simulink model "SIFT_final"  (R2015a)
settings: Solver=ode45  StartTime=0.0  StopTime=10.0  RelTol=1e-3
InitFcn:
  | %% DSPBuilder Start
  | alt_dspbuilder_update_model(bdroot)
  | %% DSPBuilder End
libraries: allblocks_alteradspbuilder2 x1826
(part 5 of 24)

== system SIFT_final/SIFT/Calculate_descriptor/hist_bin/Line_buffer_5x5_1 ==
  dataIn : Inport
  clken : Inport  Port=2
  Delay : allblocks_alteradspbuilder2/Delay  pipeline=1  pipeline_display=1  ClockPhase=1  use_ena=on  use_sclr=off  allowFloatingPointOverride=on  logOutputs=off  logFile=C:\Users\ASUS\Desktop\final_sift_fpga\tb_SIFT_detection_feature\SIFT%5Fdetection%5Ffeature_calculate%5Fdescriptor_hist%5Fbin_Line%5Fbuffer%5F5x5%5F1_Delay.fixedpointlog  use_init=off  reset_value=1
  Delay1 : allblocks_alteradspbuilder2/Delay  pipeline=1  pipeline_display=1  ClockPhase=1  use_ena=on  use_sclr=off  allowFloatingPointOverride=on  logOutputs=off  logFile=C:\Users\ASUS\Desktop\final_sift_fpga\tb_SIFT_detection_feature\SIFT%5Fdetection%5Ffeature_calculate%5Fdescriptor_hist%5Fbin_Line%5Fbuffer%5F5x5%5F1_Delay1.fixedpointlog  use_init=off  reset_value=1
  Delay10 : allblocks_alteradspbuilder2/Delay  pipeline=1  pipeline_display=1  ClockPhase=1  use_ena=on  use_sclr=off  allowFloatingPointOverride=on  logOutputs=off  logFile=C:\Users\ASUS\Desktop\final_sift_fpga\tb_SIFT_detection_feature\SIFT%5Fdetection%5Ffeature_calculate%5Fdescriptor_hist%5Fbin_Line%5Fbuffer%5F5x5%5F1_Delay10.fixedpointlog  use_init=off  reset_value=1
  Delay11 : allblocks_alteradspbuilder2/Delay  pipeline=1  pipeline_display=1  ClockPhase=1  use_ena=on  use_sclr=off  allowFloatingPointOverride=on  logOutputs=off  logFile=C:\Users\ASUS\Desktop\final_sift_fpga\tb_SIFT_detection_feature\SIFT%5Fdetection%5Ffeature_calculate%5Fdescriptor_hist%5Fbin_Line%5Fbuffer%5F5x5%5F1_Delay11.fixedpointlog  use_init=off  reset_value=1
  Delay12 : allblocks_alteradspbuilder2/Delay  pipeline=1  pipeline_display=1  ClockPhase=1  use_ena=on  use_sclr=off  allowFloatingPointOverride=on  logOutputs=off  logFile=C:\Users\ASUS\Desktop\final_sift_fpga\tb_SIFT_detection_feature\SIFT%5Fdetection%5Ffeature_calculate%5Fdescriptor_hist%5Fbin_Line%5Fbuffer%5F5x5%5F1_Delay12.fixedpointlog  use_init=off  reset_value=1
  Delay13 : allblocks_alteradspbuilder2/Delay  pipeline=1  pipeline_display=1  ClockPhase=1  use_ena=on  use_sclr=off  allowFloatingPointOverride=on  logOutputs=off  logFile=C:\Users\ASUS\Desktop\final_sift_fpga\tb_SIFT_detection_feature\SIFT%5Fdetection%5Ffeature_calculate%5Fdescriptor_hist%5Fbin_Line%5Fbuffer%5F5x5%5F1_Delay13.fixedpointlog  use_init=off  reset_value=1
  Delay14 : allblocks_alteradspbuilder2/Delay  pipeline=1  pipeline_display=1  ClockPhase=1  use_ena=on  use_sclr=off  allowFloatingPointOverride=on  logOutputs=off  logFile=C:\Users\ASUS\Desktop\final_sift_fpga\tb_SIFT_detection_feature\SIFT%5Fdetection%5Ffeature_calculate%5Fdescriptor_hist%5Fbin_Line%5Fbuffer%5F5x5%5F1_Delay14.fixedpointlog  use_init=off  reset_value=1
  Delay15 : allblocks_alteradspbuilder2/Delay  pipeline=1  pipeline_display=1  ClockPhase=1  use_ena=on  use_sclr=off  allowFloatingPointOverride=on  logOutputs=off  logFile=C:\Users\ASUS\Desktop\final_sift_fpga\tb_SIFT_detection_feature\SIFT%5Fdetection%5Ffeature_calculate%5Fdescriptor_hist%5Fbin_Line%5Fbuffer%5F5x5%5F1_Delay15.fixedpointlog  use_init=off  reset_value=1
  Delay16 : allblocks_alteradspbuilder2/Delay  pipeline=1  pipeline_display=1  ClockPhase=1  use_ena=on  use_sclr=off  allowFloatingPointOverride=on  logOutputs=off  logFile=C:\Users\ASUS\Desktop\final_sift_fpga\tb_SIFT_detection_feature\SIFT%5Fdetection%5Ffeature_calculate%5Fdescriptor_hist%5Fbin_Line%5Fbuffer%5F5x5%5F1_Delay16.fixedpointlog  use_init=off  reset_value=1
  Delay17 : allblocks_alteradspbuilder2/Delay  pipeline=1  pipeline_display=1  ClockPhase=1  use_ena=on  use_sclr=off  allowFloatingPointOverride=on  logOutputs=off  logFile=C:\Users\ASUS\Desktop\final_sift_fpga\tb_SIFT_detection_feature\SIFT%5Fdetection%5Ffeature_calculate%5Fdescriptor_hist%5Fbin_Line%5Fbuffer%5F5x5%5F1_Delay17.fixedpointlog  use_init=off  reset_value=1
  Delay18 : allblocks_alteradspbuilder2/Delay  pipeline=1  pipeline_display=1  ClockPhase=1  use_ena=on  use_sclr=off  allowFloatingPointOverride=on  logOutputs=off  logFile=C:\Users\ASUS\Desktop\final_sift_fpga\tb_SIFT_detection_feature\SIFT%5Fdetection%5Ffeature_calculate%5Fdescriptor_hist%5Fbin_Line%5Fbuffer%5F5x5%5F1_Delay18.fixedpointlog  use_init=off  reset_value=1
  Delay19 : allblocks_alteradspbuilder2/Delay  pipeline=1  pipeline_display=1  ClockPhase=1  use_ena=on  use_sclr=off  allowFloatingPointOverride=on  logOutputs=off  logFile=C:\Users\ASUS\Desktop\final_sift_fpga\tb_SIFT_detection_feature\SIFT%5Fdetection%5Ffeature_calculate%5Fdescriptor_hist%5Fbin_Line%5Fbuffer%5F5x5%5F1_Delay19.fixedpointlog  use_init=off  reset_value=1
  Delay2 : allblocks_alteradspbuilder2/Delay  pipeline=1  pipeline_display=1  ClockPhase=1  use_ena=on  use_sclr=off  allowFloatingPointOverride=on  logOutputs=off  logFile=C:\Users\ASUS\Desktop\final_sift_fpga\tb_SIFT_detection_feature\SIFT%5Fdetection%5Ffeature_calculate%5Fdescriptor_hist%5Fbin_Line%5Fbuffer%5F5x5%5F1_Delay2.fixedpointlog  use_init=off  reset_value=1
  Delay20 : allblocks_alteradspbuilder2/Delay  pipeline=1  pipeline_display=1  ClockPhase=1  use_ena=on  use_sclr=off  allowFloatingPointOverride=on  logOutputs=off  logFile=C:\Users\ASUS\Desktop\final_sift_fpga\tb_SIFT_detection_feature\SIFT%5Fdetection%5Ffeature_calculate%5Fdescriptor_hist%5Fbin_Line%5Fbuffer%5F5x5%5F1_Delay20.fixedpointlog  use_init=off  reset_value=1
  Delay21 : allblocks_alteradspbuilder2/Delay  pipeline=16  pipeline_display=16  ClockPhase=1  use_ena=on  use_sclr=off  allowFloatingPointOverride=on  logOutputs=off  logFile=C:\Users\ASUS\Desktop\final_sift_fpga\tb_SIFT_detection_feature\SIFT%5Fdetection%5Ffeature_calculate%5Fdescriptor_hist%5Fbin_Line%5Fbuffer%5F5x5%5F1_Delay21.fixedpointlog  use_init=off  reset_value=1
  Delay22 : allblocks_alteradspbuilder2/Delay  pipeline=16  pipeline_display=16  ClockPhase=1  use_ena=on  use_sclr=off  allowFloatingPointOverride=on  logOutputs=off  logFile=C:\Users\ASUS\Desktop\final_sift_fpga\tb_SIFT_detection_feature\SIFT%5Fdetection%5Ffeature_calculate%5Fdescriptor_hist%5Fbin_Line%5Fbuffer%5F5x5%5F1_Delay22.fixedpointlog  use_init=off  reset_value=1
  Delay23 : allblocks_alteradspbuilder2/Delay  pipeline=16  pipeline_display=16  ClockPhase=1  use_ena=on  use_sclr=off  allowFloatingPointOverride=on  logOutputs=off  logFile=C:\Users\ASUS\Desktop\final_sift_fpga\tb_SIFT_detection_feature\SIFT%5Fdetection%5Ffeature_calculate%5Fdescriptor_hist%5Fbin_Line%5Fbuffer%5F5x5%5F1_Delay23.fixedpointlog  use_init=off  reset_value=1
  Delay24 : allblocks_alteradspbuilder2/Delay  pipeline=16  pipeline_display=16  ClockPhase=1  use_ena=on  use_sclr=off  allowFloatingPointOverride=on  logOutputs=off  logFile=C:\Users\ASUS\Desktop\final_sift_fpga\tb_SIFT_detection_feature\SIFT%5Fdetection%5Ffeature_calculate%5Fdescriptor_hist%5Fbin_Line%5Fbuffer%5F5x5%5F1_Delay24.fixedpointlog  use_init=off  reset_value=1
  Delay25 : allblocks_alteradspbuilder2/Delay  pipeline=16  pipeline_display=16  ClockPhase=1  use_ena=on  use_sclr=off  allowFloatingPointOverride=on  logOutputs=off  logFile=C:\Users\ASUS\Desktop\final_sift_fpga\tb_SIFT_detection_feature\SIFT%5Fdetection%5Ffeature_calculate%5Fdescriptor_hist%5Fbin_Line%5Fbuffer%5F5x5%5F1_Delay25.fixedpointlog  use_init=off  reset_value=1
  Delay26 : allblocks_alteradspbuilder2/Delay  pipeline=16  pipeline_display=16  ClockPhase=1  use_ena=on  use_sclr=off  allowFloatingPointOverride=on  logOutputs=off  logFile=C:\Users\ASUS\Desktop\final_sift_fpga\tb_SIFT_detection_feature\SIFT%5Fdetection%5Ffeature_calculate%5Fdescriptor_hist%5Fbin_Line%5Fbuffer%5F5x5%5F1_Delay26.fixedpointlog  use_init=off  reset_value=1
  Delay27 : allblocks_alteradspbuilder2/Delay  pipeline=16  pipeline_display=16  ClockPhase=1  use_ena=on  use_sclr=off  allowFloatingPointOverride=on  logOutputs=off  logFile=C:\Users\ASUS\Desktop\final_sift_fpga\tb_SIFT_detection_feature\SIFT%5Fdetection%5Ffeature_calculate%5Fdescriptor_hist%5Fbin_Line%5Fbuffer%5F5x5%5F1_Delay27.fixedpointlog  use_init=off  reset_value=1
  Delay28 : allblocks_alteradspbuilder2/Delay  pipeline=16  pipeline_display=16  ClockPhase=1  use_ena=on  use_sclr=off  allowFloatingPointOverride=on  logOutputs=off  logFile=C:\Users\ASUS\Desktop\final_sift_fpga\tb_SIFT_detection_feature\SIFT%5Fdetection%5Ffeature_calculate%5Fdescriptor_hist%5Fbin_Line%5Fbuffer%5F5x5%5F1_Delay28.fixedpointlog  use_init=off  reset_value=1
  Delay29 : allblocks_alteradspbuilder2/Delay  pipeline=16  pipeline_display=16  ClockPhase=1  use_ena=on  use_sclr=off  allowFloatingPointOverride=on  logOutputs=off  logFile=C:\Users\ASUS\Desktop\final_sift_fpga\tb_SIFT_detection_feature\SIFT%5Fdetection%5Ffeature_calculate%5Fdescriptor_hist%5Fbin_Line%5Fbuffer%5F5x5%5F1_Delay29.fixedpointlog  use_init=off  reset_value=1
  Delay3 : allblocks_alteradspbuilder2/Delay  pipeline=1  pipeline_display=1  ClockPhase=1  use_ena=on  use_sclr=off  allowFloatingPointOverride=on  logOutputs=off  logFile=C:\Users\ASUS\Desktop\final_sift_fpga\tb_SIFT_detection_feature\SIFT%5Fdetection%5Ffeature_calculate%5Fdescriptor_hist%5Fbin_Line%5Fbuffer%5F5x5%5F1_Delay3.fixedpointlog  use_init=off  reset_value=1
  Delay30 : allblocks_alteradspbuilder2/Delay  pipeline=16  pipeline_display=16  ClockPhase=1  use_ena=on  use_sclr=off  allowFloatingPointOverride=on  logOutputs=off  logFile=C:\Users\ASUS\Desktop\final_sift_fpga\tb_SIFT_detection_feature\SIFT%5Fdetection%5Ffeature_calculate%5Fdescriptor_hist%5Fbin_Line%5Fbuffer%5F5x5%5F1_Delay30.fixedpointlog  use_init=off  reset_value=1
  Delay31 : allblocks_alteradspbuilder2/Delay  pipeline=16  pipeline_display=16  ClockPhase=1  use_ena=on  use_sclr=off  allowFloatingPointOverride=on  logOutputs=off  logFile=C:\Users\ASUS\Desktop\final_sift_fpga\tb_SIFT_detection_feature\SIFT%5Fdetection%5Ffeature_calculate%5Fdescriptor_hist%5Fbin_Line%5Fbuffer%5F5x5%5F1_Delay31.fixedpointlog  use_init=off  reset_value=1
  Delay32 : allblocks_alteradspbuilder2/Delay  pipeline=16  pipeline_display=16  ClockPhase=1  use_ena=on  use_sclr=off  allowFloatingPointOverride=on  logOutputs=off  logFile=C:\Users\ASUS\Desktop\final_sift_fpga\tb_SIFT_detection_feature\SIFT%5Fdetection%5Ffeature_calculate%5Fdescriptor_hist%5Fbin_Line%5Fbuffer%5F5x5%5F1_Delay32.fixedpointlog  use_init=off  reset_value=1
  Delay33 : allblocks_alteradspbuilder2/Delay  pipeline=16  pipeline_display=16  ClockPhase=1  use_ena=on  use_sclr=off  allowFloatingPointOverride=on  logOutputs=off  logFile=C:\Users\ASUS\Desktop\final_sift_fpga\tb_SIFT_detection_feature\SIFT%5Fdetection%5Ffeature_calculate%5Fdescriptor_hist%5Fbin_Line%5Fbuffer%5F5x5%5F1_Delay33.fixedpointlog  use_init=off  reset_value=1
  Delay34 : allblocks_alteradspbuilder2/Delay  pipeline=16  pipeline_display=16  ClockPhase=1  use_ena=on  use_sclr=off  allowFloatingPointOverride=on  logOutputs=off  logFile=C:\Users\ASUS\Desktop\final_sift_fpga\tb_SIFT_detection_feature\SIFT%5Fdetection%5Ffeature_calculate%5Fdescriptor_hist%5Fbin_Line%5Fbuffer%5F5x5%5F1_Delay34.fixedpointlog  use_init=off  reset_value=1
  Delay35 : allblocks_alteradspbuilder2/Delay  pipeline=16  pipeline_display=16  ClockPhase=1  use_ena=on  use_sclr=off  allowFloatingPointOverride=on  logOutputs=off  logFile=C:\Users\ASUS\Desktop\final_sift_fpga\tb_SIFT_detection_feature\SIFT%5Fdetection%5Ffeature_calculate%5Fdescriptor_hist%5Fbin_Line%5Fbuffer%5F5x5%5F1_Delay35.fixedpointlog  use_init=off  reset_value=1
  Delay36 : allblocks_alteradspbuilder2/Delay  pipeline=16  pipeline_display=16  ClockPhase=1  use_ena=on  use_sclr=off  allowFloatingPointOverride=on  logOutputs=off  logFile=C:\Users\ASUS\Desktop\final_sift_fpga\tb_SIFT_detection_feature\SIFT%5Fdetection%5Ffeature_calculate%5Fdescriptor_hist%5Fbin_Line%5Fbuffer%5F5x5%5F1_Delay36.fixedpointlog  use_init=off  reset_value=1
  Delay37 : allblocks_alteradspbuilder2/Delay  pipeline=16  pipeline_display=16  ClockPhase=1  use_ena=on  use_sclr=off  allowFloatingPointOverride=on  logOutputs=off  logFile=C:\Users\ASUS\Desktop\final_sift_fpga\tb_SIFT_detection_feature\SIFT%5Fdetection%5Ffeature_calculate%5Fdescriptor_hist%5Fbin_Line%5Fbuffer%5F5x5%5F1_Delay37.fixedpointlog  use_init=off  reset_value=1
  Delay38 : allblocks_alteradspbuilder2/Delay  pipeline=16  pipeline_display=16  ClockPhase=1  use_ena=on  use_sclr=off  allowFloatingPointOverride=on  logOutputs=off  logFile=C:\Users\ASUS\Desktop\final_sift_fpga\tb_SIFT_detection_feature\SIFT%5Fdetection%5Ffeature_calculate%5Fdescriptor_hist%5Fbin_Line%5Fbuffer%5F5x5%5F1_Delay38.fixedpointlog  use_init=off  reset_value=1
  Delay39 : allblocks_alteradspbuilder2/Delay  pipeline=16  pipeline_display=16  ClockPhase=1  use_ena=on  use_sclr=off  allowFloatingPointOverride=on  logOutputs=off  logFile=C:\Users\ASUS\Desktop\final_sift_fpga\tb_SIFT_detection_feature\SIFT%5Fdetection%5Ffeature_calculate%5Fdescriptor_hist%5Fbin_Line%5Fbuffer%5F5x5%5F1_Delay39.fixedpointlog  use_init=off  reset_value=1
  Delay4 : allblocks_alteradspbuilder2/Delay  pipeline=1  pipeline_display=1  ClockPhase=1  use_ena=on  use_sclr=off  allowFloatingPointOverride=on  logOutputs=off  logFile=C:\Users\ASUS\Desktop\final_sift_fpga\tb_SIFT_detection_feature\SIFT%5Fdetection%5Ffeature_calculate%5Fdescriptor_hist%5Fbin_Line%5Fbuffer%5F5x5%5F1_Delay4.fixedpointlog  use_init=off  reset_value=1
  Delay40 : allblocks_alteradspbuilder2/Delay  pipeline=16  pipeline_display=16  ClockPhase=1  use_ena=on  use_sclr=off  allowFloatingPointOverride=on  logOutputs=off  logFile=C:\Users\ASUS\Desktop\final_sift_fpga\tb_SIFT_detection_feature\SIFT%5Fdetection%5Ffeature_calculate%5Fdescriptor_hist%5Fbin_Line%5Fbuffer%5F5x5%5F1_Delay40.fixedpointlog  use_init=off  reset_value=1
  Delay41 : allblocks_alteradspbuilder2/Delay  pipeline=16  pipeline_display=16  ClockPhase=1  use_ena=on  use_sclr=off  allowFloatingPointOverride=on  logOutputs=off  logFile=C:\Users\ASUS\Desktop\final_sift_fpga\tb_SIFT_detection_feature\SIFT%5Fdetection%5Ffeature_calculate%5Fdescriptor_hist%5Fbin_Line%5Fbuffer%5F5x5%5F1_Delay41.fixedpointlog  use_init=off  reset_value=1
  Delay42 : allblocks_alteradspbuilder2/Delay  pipeline=16  pipeline_display=16  ClockPhase=1  use_ena=on  use_sclr=off  allowFloatingPointOverride=on  logOutputs=off  logFile=C:\Users\ASUS\Desktop\final_sift_fpga\tb_SIFT_detection_feature\SIFT%5Fdetection%5Ffeature_calculate%5Fdescriptor_hist%5Fbin_Line%5Fbuffer%5F5x5%5F1_Delay42.fixedpointlog  use_init=off  reset_value=1
  Delay43 : allblocks_alteradspbuilder2/Delay  pipeline=16  pipeline_display=16  ClockPhase=1  use_ena=on  use_sclr=off  allowFloatingPointOverride=on  logOutputs=off  logFile=C:\Users\ASUS\Desktop\final_sift_fpga\tb_SIFT_detection_feature\SIFT%5Fdetection%5Ffeature_calculate%5Fdescriptor_hist%5Fbin_Line%5Fbuffer%5F5x5%5F1_Delay43.fixedpointlog  use_init=off  reset_value=1
  Delay44 : allblocks_alteradspbuilder2/Delay  pipeline=16  pipeline_display=16  ClockPhase=1  use_ena=on  use_sclr=off  allowFloatingPointOverride=on  logOutputs=off  logFile=C:\Users\ASUS\Desktop\final_sift_fpga\tb_SIFT_detection_feature\SIFT%5Fdetection%5Ffeature_calculate%5Fdescriptor_hist%5Fbin_Line%5Fbuffer%5F5x5%5F1_Delay44.fixedpointlog  use_init=off  reset_value=1
  Delay45 : allblocks_alteradspbuilder2/Delay  pipeline=16  pipeline_display=16  ClockPhase=1  use_ena=on  use_sclr=off  allowFloatingPointOverride=on  logOutputs=off  logFile=C:\Users\ASUS\Desktop\final_sift_fpga\tb_SIFT_detection_feature\SIFT%5Fdetection%5Ffeature_calculate%5Fdescriptor_hist%5Fbin_Line%5Fbuffer%5F5x5%5F1_Delay45.fixedpointlog  use_init=off  reset_value=1
  Delay5 : allblocks_alteradspbuilder2/Delay  pipeline=1  pipeline_display=1  ClockPhase=1  use_ena=on  use_sclr=off  allowFloatingPointOverride=on  logOutputs=off  logFile=C:\Users\ASUS\Desktop\final_sift_fpga\tb_SIFT_detection_feature\SIFT%5Fdetection%5Ffeature_calculate%5Fdescriptor_hist%5Fbin_Line%5Fbuffer%5F5x5%5F1_Delay5.fixedpointlog  use_init=off  reset_value=1
  Delay6 : allblocks_alteradspbuilder2/Delay  pipeline=1  pipeline_display=1  ClockPhase=1  use_ena=on  use_sclr=off  allowFloatingPointOverride=on  logOutputs=off  logFile=C:\Users\ASUS\Desktop\final_sift_fpga\tb_SIFT_detection_feature\SIFT%5Fdetection%5Ffeature_calculate%5Fdescriptor_hist%5Fbin_Line%5Fbuffer%5F5x5%5F1_Delay6.fixedpointlog  use_init=off  reset_value=1
  Delay7 : allblocks_alteradspbuilder2/Delay  pipeline=1  pipeline_display=1  ClockPhase=1  use_ena=on  use_sclr=off  allowFloatingPointOverride=on  logOutputs=off  logFile=C:\Users\ASUS\Desktop\final_sift_fpga\tb_SIFT_detection_feature\SIFT%5Fdetection%5Ffeature_calculate%5Fdescriptor_hist%5Fbin_Line%5Fbuffer%5F5x5%5F1_Delay7.fixedpointlog  use_init=off  reset_value=1
  Delay8 : allblocks_alteradspbuilder2/Delay  pipeline=1  pipeline_display=1  ClockPhase=1  use_ena=on  use_sclr=off  allowFloatingPointOverride=on  logOutputs=off  logFile=C:\Users\ASUS\Desktop\final_sift_fpga\tb_SIFT_detection_feature\SIFT%5Fdetection%5Ffeature_calculate%5Fdescriptor_hist%5Fbin_Line%5Fbuffer%5F5x5%5F1_Delay8.fixedpointlog  use_init=off  reset_value=1
  Delay9 : allblocks_alteradspbuilder2/Delay  pipeline=1  pipeline_display=1  ClockPhase=1  use_ena=on  use_sclr=off  allowFloatingPointOverride=on  logOutputs=off  logFile=C:\Users\ASUS\Desktop\final_sift_fpga\tb_SIFT_detection_feature\SIFT%5Fdetection%5Ffeature_calculate%5Fdescriptor_hist%5Fbin_Line%5Fbuffer%5F5x5%5F1_Delay9.fixedpointlog  use_init=off  reset_value=1
  Memory Delay : allblocks_alteradspbuilder2/Memory Delay  BusType=Unsigned Integer  bwl=8  bwr=0  pipeline=636  pipeline_display=636  ram_type=AUTO  use_ena=on  use_sclr=off  allowFloatingPointOverride=on  logOutputs=off  logFile=C:\Users\ASUS\Desktop\final_sift_fpga\tb_SIFT_detection_feature\SIFT%5Fdetection%5Ffeature_calculate%5Fdescriptor_hist%5Fbin_Line%5Fbuffer%5F5x5%5F1_Memory+Delay.fixedpointlog
  Memory Delay1 : allblocks_alteradspbuilder2/Memory Delay  BusType=Unsigned Integer  bwl=8  bwr=0  pipeline=636  pipeline_display=636  ram_type=AUTO  use_ena=on  use_sclr=off  allowFloatingPointOverride=on  logOutputs=off  logFile=C:\Users\ASUS\Desktop\final_sift_fpga\tb_SIFT_detection_feature\SIFT%5Fdetection%5Ffeature_calculate%5Fdescriptor_hist%5Fbin_Line%5Fbuffer%5F5x5%5F1_Memory+Delay1.fixedpointlog
  Memory Delay2 : allblocks_alteradspbuilder2/Memory Delay  BusType=Unsigned Integer  bwl=8  bwr=0  pipeline=636  pipeline_display=636  ram_type=AUTO  use_ena=on  use_sclr=off  allowFloatingPointOverride=on  logOutputs=off  logFile=C:\Users\ASUS\Desktop\final_sift_fpga\tb_SIFT_detection_feature\SIFT%5Fdetection%5Ffeature_calculate%5Fdescriptor_hist%5Fbin_Line%5Fbuffer%5F5x5%5F1_Memory+Delay2.fixedpointlog
  Memory Delay3 : allblocks_alteradspbuilder2/Memory Delay  BusType=Unsigned Integer  bwl=8  bwr=0  pipeline=636  pipeline_display=636  ram_type=AUTO  use_ena=on  use_sclr=off  allowFloatingPointOverride=on  logOutputs=off  logFile=C:\Users\ASUS\Desktop\final_sift_fpga\tb_SIFT_detection_feature\SIFT%5Fdetection%5Ffeature_calculate%5Fdescriptor_hist%5Fbin_Line%5Fbuffer%5F5x5%5F1_Memory+Delay3.fixedpointlog
  Out00 : Outport
  Out01 : Outport  Port=2
  Out02 : Outport  Port=3
  Out03 : Outport  Port=4
  Out04 : Outport  Port=5
  Out10 : Outport  Port=6
  Out11 : Outport  Port=7
  Out12 : Outport  Port=8
  Out13 : Outport  Port=9
  Out14 : Outport  Port=10
  Out20 : Outport  Port=11
  Out21 : Outport  Port=12
  Out22 : Outport  Port=13
  Out23 : Outport  Port=14
  Out24 : Outport  Port=15
  Out30 : Outport  Port=16
  Out31 : Outport  Port=17
  Out32 : Outport  Port=18
  Out33 : Outport  Port=19
  Out34 : Outport  Port=20
  Out40 : Outport  Port=21
  Out41 : Outport  Port=22
  Out42 : Outport  Port=23
  Out43 : Outport  Port=24
  Out44 : Outport  Port=25
  wires:
  [clken] -> Delay11/2
  Delay11/1 -> [data_23], Delay12/1
  [clken] -> Delay12/2
  [clken] -> Delay10/2
  Delay8/1 -> Memory Delay1/1, [data_14]
  [clken] -> Memory Delay1/2
  Delay9/1 -> [data_21], Delay10/1
  Memory Delay1/1 -> [data_20], Delay9/1
  Delay10/1 -> [data_22], Delay11/1
  [clken] -> Delay9/2
  [clken] -> Delay4/2
  Delay/1 -> [data_00], Delay1/1
  [clken] -> Delay1/2
  [clken] -> Delay/2
  [data_in] -> Delay/1
  [clken] -> Delay2/2
  Delay2/1 -> [data_02], Delay3/1
  Delay1/1 -> [data_01], Delay2/1
  [clken] -> Delay3/2
  clken/1 -> [clken]
  dataIn/1 -> [data_in]
  Delay4/1 -> Memory Delay/1, [data_04]
  [clken] -> Memory Delay/2
  Delay12/1 -> [data_24], Memory Delay2/1
  [clken] -> Memory Delay2/2
  Memory Delay2/1 -> [data_30], Delay16/1
  [clken] -> Delay16/2
  [clken] -> Delay14/2
  [clken] -> Delay15/2
  [clken] -> Memory Delay3/2
  Delay17/1 -> [data_32], Delay18/1
  Delay18/1 -> [data_33], Delay19/1
  Memory Delay3/1 -> [data_40], Delay20/1
  [clken] -> Delay20/2
  [clken] -> Delay19/2
  Delay13/1 -> [data_42], Delay14/1
  Delay19/1 -> Memory Delay3/1, [data_34]
  Delay14/1 -> [data_43], Delay15/1
  Delay15/1 -> [data_44]
  [clken] -> Delay17/2
  [clken] -> Delay18/2
  [clken] -> Delay13/2
  Delay16/1 -> [data_31], Delay17/1
  Delay20/1 -> [data_41], Delay13/1
  Memory Delay/1 -> [data_10], Delay5/1
  [clken] -> Delay7/2
  [clken] -> Delay6/2
  Delay5/1 -> [data_11], Delay6/1
  [clken] -> Delay8/2
  [clken] -> Delay5/2
  Delay7/1 -> [data_13], Delay8/1
  Delay6/1 -> [data_12], Delay7/1
  Delay3/1 -> [data_03], Delay4/1
  [data_03] -> Delay24/1
  [data_04] -> Delay25/1
  [data_02] -> Delay23/1
  [data_32] -> Delay38/1
  [data_44] -> Delay45/1
  [data_31] -> Delay37/1
  [data_40] -> Delay41/1
  [data_34] -> Delay40/1
  [data_30] -> Delay36/1
  [data_33] -> Delay39/1
  [data_43] -> Delay44/1
  [data_42] -> Delay43/1
  [data_41] -> Delay42/1
  [data_01] -> Delay22/1
  [data_00] -> Delay21/1
  [data_21] -> Delay32/1
  [data_20] -> Delay31/1
  [data_23] -> Delay34/1
  [data_22] -> Delay33/1
  [data_24] -> Delay35/1
  [data_10] -> Delay26/1
  [data_11] -> Delay27/1
  [data_12] -> Delay28/1
  [data_13] -> Delay29/1
  [data_14] -> Delay30/1
  Delay21/1 -> Out00/1
  Delay22/1 -> Out01/1
  Delay23/1 -> Out02/1
  Delay24/1 -> Out03/1
  Delay25/1 -> Out04/1
  Delay26/1 -> Out10/1
  Delay27/1 -> Out11/1
  Delay28/1 -> Out12/1
  Delay29/1 -> Out13/1
  Delay30/1 -> Out14/1
  Delay31/1 -> Out20/1
  Delay32/1 -> Out21/1
  Delay33/1 -> Out22/1
  Delay34/1 -> Out23/1
  Delay35/1 -> Out24/1
  [clken] -> Delay21/2, Delay35/2, Delay34/2, Delay33/2, Delay32/2, Delay31/2, Delay30/2, Delay29/2, Delay28/2, Delay27/2, Delay26/2, Delay25/2, Delay24/2, Delay23/2, Delay22/2
  Delay36/1 -> Out30/1
  Delay37/1 -> Out31/1
  Delay38/1 -> Out32/1
  Delay39/1 -> Out33/1
  Delay40/1 -> Out34/1
  Delay41/1 -> Out40/1
  Delay42/1 -> Out41/1
  Delay43/1 -> Out42/1
  Delay44/1 -> Out43/1
  Delay45/1 -> Out44/1
  [clken] -> Delay45/2, Delay44/2, Delay43/2, Delay42/2, Delay41/2, Delay40/2, Delay39/2, Delay38/2, Delay37/2, Delay36/2
